simulink model "exercise_fixedpoint"  (R2012b)
settings: Solver=VariableStepDiscrete  StartTime=0.0  StopTime=1  RelTol=1e-3
settings Model: Creator=morgy  LastModifiedBy=morgy

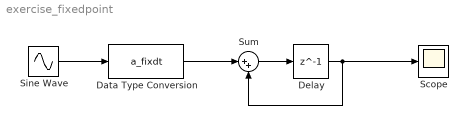
== system exercise_fixedpoint ==
  Data Type Conversion : DataTypeConversion  OutDataTypeStr=a_fixdt  LockScale=on
  Delay : Delay  DelayLength=1  InitialCondition=0
  Scope : Scope
  Sine Wave : Sin  Frequency=2*pi*100  SampleTime=1/48000
  Sum : Sum  Inputs=|++  AccumDataTypeStr=a_fixdt
  wires:
  Sum/1 -> Delay/1
  Sine Wave/1 -> Data Type Conversion/1
  Delay/1 -> Scope/1, Sum/2
  Data Type Conversion/1 -> Sum/1
